simulink model "T_TEM_matched"  (R2015a)
settings: Solver=ode3  StartTime=0.0  StopTime=94  FixedStep=1  RelTol=1e-3
libraries: LU_TEG x1
settings Model: Creator=lansong7  LastModifiedBy=ttsl6

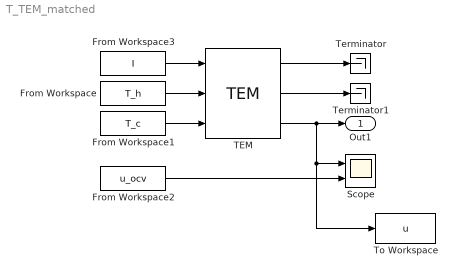
== system T_TEM_matched ==
  From Workspace : FromWorkspace  VariableName=T_h  SampleTime=0
  From Workspace1 : FromWorkspace  VariableName=T_c  SampleTime=0
  From Workspace2 : FromWorkspace  VariableName=u_ocv  SampleTime=0
  From Workspace3 : FromWorkspace  VariableName=I  SampleTime=0
  Scope : Scope  NumInputPorts=2
      settings: TimeRange=159  YMin=300~0  YMax=380~7
  TEM : LU_TEG/TEM  l=l  l_cw=l_cw  f=f  a=a  n=n  Tune_tr=Tune_tr  Tune_er=Tune_er  ct1=ct1  ct2=ct2
  Terminator : Terminator
  Terminator1 : Terminator
  To Workspace : ToWorkspace  VariableName=u  SaveFormat=Structure With Time  SampleTime=-1
  Out1 : Outport
  wires:
  From Workspace/1 -> TEM/2
  From Workspace1/1 -> TEM/3
  From Workspace3/1 -> TEM/1
  TEM/2 -> Terminator1/1
  TEM/1 -> Terminator/1
  From Workspace2/1 -> Scope/2
  TEM/3 -> Scope/1, To Workspace/1, Out1/1
